simulink model "TST_AdvancedStateflowLoops"  (Simulink 10.0)
settings: Solver=FixedStepDiscrete  StartTime=0.0  StopTime=10.0  FixedStep=0.02  RelTol=1e-3  EnableMultiTasking=on
settings Model: Creator=kharthforeign  LastModifiedBy=unknown
settings DataIOCC: LimitDataPoints=on  SignalLoggingSaveFormat=ModelDataLogs  SaveOutput=off  SignalLogging=off  SaveTime=off
settings OptimizationCC: BlockReduction=off  ConditionallyExecuteInputs=off  OptimizeBlockIOStorage=off  BufferReuse=off  GlobalBufferReuse=off  ExpressionFolding=off  ExpressionDepthLimit=2147483647  LocalBlockOutputs=off  InitFltsAndDblsToZero=on  OptimizeDataStoreBuffers=off  BusAssignmentInplaceUpdate=off
settings DebuggingCC: SolverPrmCheckMsg=warning  FcnCallInpInsideContextMsg=warning  StateNameClashWarn=warning
settings SFSimCC: SimParseCustomCode=off
settings GRTTargetCC: GeneratePreprocessorConditionals=Disable all
settings ConfigComp: CovExternalEMLEnable=off

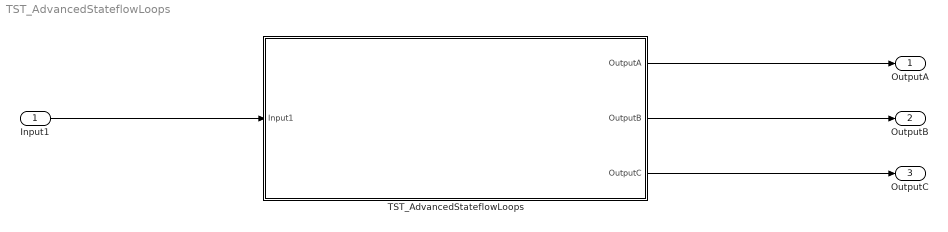
== system TST_AdvancedStateflowLoops ==
  Input1 : Inport  OutDataTypeStr=uint32  BusOutputAsStruct=on
  TST_AdvancedStateflowLoops : Subsystem  TreatAsAtomicUnit=on
  OutputA : Outport  OutDataTypeStr=double  PortDimensions=1
  OutputB : Outport  Port=2  OutDataTypeStr=double  PortDimensions=1
  OutputC : Outport  Port=3  OutDataTypeStr=double  PortDimensions=1
  wires:
  Input1/1 -> TST_AdvancedStateflowLoops/1(Input1)
  TST_AdvancedStateflowLoops/1(OutputA) -> OutputA/1
  TST_AdvancedStateflowLoops/2(OutputB) -> OutputB/1
  TST_AdvancedStateflowLoops/3(OutputC) -> OutputC/1

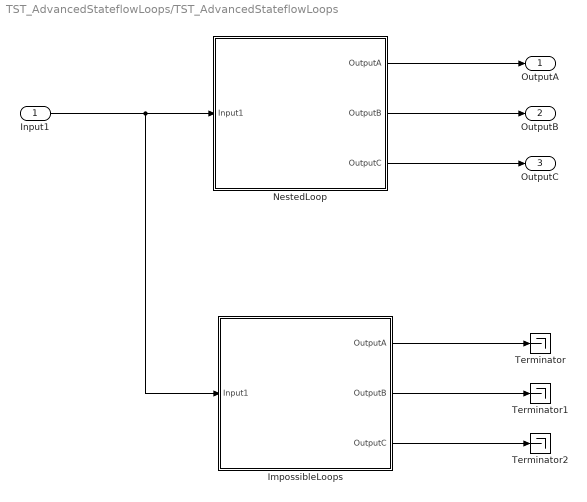
== system TST_AdvancedStateflowLoops/TST_AdvancedStateflowLoops ==
  Input1 : Inport  OutDataTypeStr=uint32  BusOutputAsStruct=on
  ImpossibleLoops : Stateflow chart  TreatAsAtomicUnit=on
  NestedLoop : Stateflow chart  TreatAsAtomicUnit=on
  Terminator : Terminator
  Terminator1 : Terminator
  Terminator2 : Terminator
  OutputA : Outport  OutDataTypeStr=double  PortDimensions=1
  OutputB : Outport  Port=2  OutDataTypeStr=double  PortDimensions=1
  OutputC : Outport  Port=3  OutDataTypeStr=double  PortDimensions=1
  wires:
  NestedLoop/1(OutputA) -> OutputA/1
  NestedLoop/2(OutputB) -> OutputB/1
  NestedLoop/3(OutputC) -> OutputC/1
  Input1/1 -> NestedLoop/1(Input1), ImpossibleLoops/1(Input1)
  ImpossibleLoops/1(OutputA) -> Terminator/1
  ImpossibleLoops/2(OutputB) -> Terminator1/1
  ImpossibleLoops/3(OutputC) -> Terminator2/1

== stateflow chart TST_AdvancedStateflowLoops/NestedLoop ==
  note: demonstrate loop nested inside another loop
  (default) -> (junction 13) : %default
  (junction 13) -> (junction 12) [order 2] : %else to A
  (junction 14) -> (junction 13) : %loop1.4
  (junction 13) -> (junction 15) [order 1] : [A]{OutputA = 1;}%loop1.1
  (junction 16) -> (junction 14) [order 2] : %else to B, loop1.3
  (junction 16) -> (junction 16) [order 1] : [B]{OutputB = 1;} %loop 2.1
  (junction 15) -> (junction 16) : %loop1.2
  data: Input1 input uint32; OutputA output double =1; OutputB output double =2; OutputC output double =3; Local local uint32 =0; A local boolean; B local boolean; C local boolean

== stateflow chart TST_AdvancedStateflowLoops/ImpossibleLoops ==
  note: Designing something like this is probably
      | not a good idea!
  note: Even though the graphical presentation doesn not show this
      | well: The second loop (starting with [D] is simply nested
      | inside the first loop (starting at [A]...). Both loops share the [D] transition.
  (default) -> (junction 38) : %default
  (junction 38) -> (junction 37) [order 2] : %else to A
  (junction 41) -> (junction 38) [order 1] : [B]{OutputB = 1;}%loop1.3
  (junction 38) -> (junction 39) [order 1] : [A]{OutputA = 1;}%loop1.1
  (junction 39) -> (junction 40) [order 2] : %else to D
  (junction 42) -> (junction 39) [order 1] : [C]{OutputC = 1;}%loop2.3
  (junction 39) -> (junction 41) [order 1] : [D]%loop1.2/2.1
  (junction 41) -> (junction 42) [order 2] : %else to B/loop2.2
  (junction 42) -> (junction 43) [order 2] : %else to C
  data: Input1 input uint32; OutputA output double =1; OutputB output double =2; OutputC output double =3; Local local uint32 =0; A local boolean; B local boolean; C local boolean; D local boolean
